simulink model "Modulation_cosim"  (Simulink 6.3)
settings: Solver=FixedStepDiscrete  StartTime=0.0  StopTime=15.0  RelTol=1e-3
undefined symbols (not defined in the file): image, port_label
libraries: aldec_ahdl x3
settings Model: LastModifiedBy=arekg
settings DataIOCC: SignalLoggingName=sigsOut
settings OptimizationCC: InlineInvariantSignals=on
settings DebuggingCC: SolverPrmCheckMsg=none
settings HardwareCC: TargetUnknown=on
settings GRTTargetCC: ModelReferenceCompliant=off  MatFileLogging=off

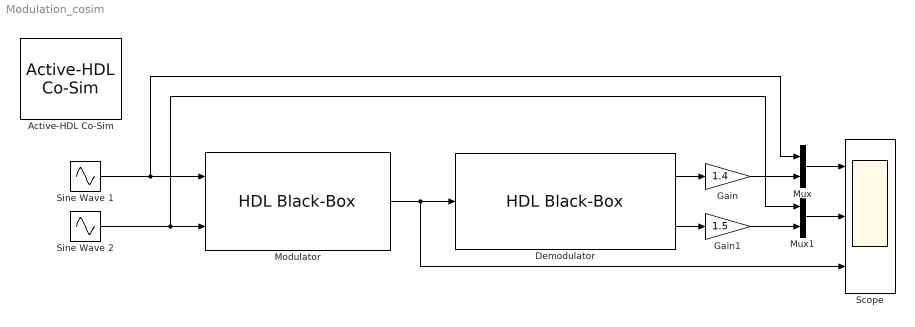
== system Modulation_cosim ==
  Active-HDL Co-Sim : aldec_ahdl/Active-HDL Co-Sim  hdl_period=1/40  hdl_tscale=sec  sys_period=1/20  sys_tscale=As In Simulator  wav_fn=mlab_cosim  wav_settings=[0,0,0,0]  dbg=off  auto_start=off  gen_tb=off  batch_sim=off  tb_fn=mlab_post_tb.log  metavalue_map=[0,0]  sim_resolution=[1,0,0]  active_page=0
  Demodulator : aldec_ahdl/HDL Black-Box  module_m=top_demodulator  ports_cfg={clk,3,1,0,0,1,8,0,0,1,0,0}{reset,5,1,0,0,1,8,0,0,1,0,0}{In1,0,31,24,24,1,0,0,0,0,0,0}{envelope,1,21,5,5,clk,0,0,0,0,0,0}{carrier,1,21,5,5,clk,0,0,0,0,0,0}  clocks={0,2,0,0.5000}  stims={1,1 0ms 0 50ms}  hdl_src=c:\My_Designs\Samples_72\Simulink_modulation\Demodulator\src\fir_32.vhd;c:\My_Designs\Samples_72\Simulink_modulation\Demodulator\src\abs.vhd;c:\My_Designs\Samples_72\Simulink_modulation\Demodulator\src\sign.vhd;c:\My_Designs\Samples_72\Simulink_modulation\Demodulator\compile\top_demodulator.vhd  block_mask=image(imread('HDLBlackBox.jpg'),'center'); disp('top_demodulator');port_label('input', 1, 'In1'); port_label('output', 1, 'envelope'); port_label('output', 2, 'carrier');  inp=[1,0,31,24]  out=[2,0,21,5,0,21,5]  sampling=[0,2]  active_page=0  param_val=0  port_in_val=0  port_out_val=0  clk_val=0  ce_val=0  config=0
  Gain : Gain  Gain=1.4
  Gain1 : Gain  Gain=1.5
  Modulator : aldec_ahdl/HDL Black-Box  module_m=mult  ports_cfg={Sin_wav1,0,16,9,9,1,0,0,0,0,0,0}{Sin_wav2,0,16,15,15,1,0,0,0,0,0,0}{Out1,1,31,24,24,2,0,0,0,0,0,0}  hdl_src=c:\My_Designs\Samples_72\Simulink_modulation\modulator\src\mult.vhd  block_mask=image(imread('HDLBlackBox.jpg'),'center'); disp('mult');port_label('input', 1, 'Sin_wav1'); port_label('input', 2, 'Sin_wav2'); port_label('output', 1, 'Out1');  inp=[2,0,16,9,0,16,15]  out=[1,0,31,24]  sampling=[0,2]  active_page=0  param_val=0  port_in_val=0  port_out_val=0  clk_val=0  ce_val=0  config=0
  Mux : Mux  Inputs=2
  Mux1 : Mux  Inputs=2
  Scope : Scope  NumInputPorts=3
      settings: TimeRange=15  YMin=0~-1.5~-40  YMax=40~1.5~40
  Sine Wave 1 : Sin  Amplitude=18  Bias=20  Frequency=0.2*(2*pi)  Phase=pi/1.3  SampleTime=1/20
  Sine Wave 2 : Sin  Amplitude=0.9  Frequency=1.18*(2*pi)  Phase=pi  SampleTime=1/20
  wires:
  Sine Wave 1/1 -> Modulator/1, Mux/1
  Sine Wave 2/1 -> Modulator/2, Mux1/1
  Modulator/1 -> Demodulator/1, Scope/3
  Mux/1 -> Scope/1
  Demodulator/1 -> Gain/1
  Gain/1 -> Mux/2
  Mux1/1 -> Scope/2
  Demodulator/2 -> Gain1/1
  Gain1/1 -> Mux1/2
